simulink model "LPV_PitchControl_TwrFA_CP_Demonstrator_Integrator_TSR"  (R2018a)
settings: Solver=FixedStepAuto  StartTime=0.0  StopTime=TMax  FixedStep=Simulation.DT  RelTol=1e-3  EnableMultiTasking=on
undefined symbols (not defined in the file or in its folder): OutList, Parameters, rpm2radps, Simulation, strmatch
libraries: dspstat3 x4, simulink_extras x1
(part 1 of 2)
settings Model: ExtModeTrigMode=oneshot  ExtModeArmWhenConnect=off  Creator=Dana Martin  LastModifiedBy=dmartin
settings DataIOCC: SaveFormat=Array  SaveOutput=off  InspectSignalLogs=on  SignalLoggingName=sigsOut  OutputTimes=[0:500]/50
settings OptimizationCC: BooleanDataType=off  ExpressionDepthLimit=2147483647  InitFltsAndDblsToZero=on  LifeSpan=inf
settings DebuggingCC: SignalRangeChecking=warning  AlgebraicLoopMsg=error  SaveWithParameterizedLinksMsg=none  UnderspecifiedInitializationDetection=Classic  MergeDetectMultiDrivingBlocksExec=none  SignalResolutionControl=TryResolveAllWithWarning  TimeAdjustmentMsg=warning  MultiTaskDSMMsg=warning  MultiTaskCondExecSysMsg=warning  ParameterUnderflowMsg=warning  UnderSpecifiedDataTypeMsg=warning  UnnecessaryDatatypeConvMsg=warning  VectorMatrixConversionMsg=warning  FcnCallInpInsideContextMsg=warning  SignalLabelMismatchMsg=warning  SFcnCompatibilityMsg=warning  UniqueDataStoreMsg=warning  AllowSymbolicDim=off  ModelReferenceIOMsg=warning  ModelReferenceVersionMismatchMessage=warning  ModelReferenceIOMismatchMessage=warning  StateNameClashWarn=warning  StrictBusMsg=WarnOnBusTreatedAsVector  NonBusSignalsTreatedAsBus=warning  SFUnexpectedBacktrackingDiag=warning  SFNoUnconditionalDefaultTransitionDiag=warning  SFExecutionAtInitializationDiag=none
settings HardwareCC: ProdBitPerPointer=32  ProdBitPerSizeT=32  ProdBitPerPtrDiffT=32  ProdLargestAtomicFloat=None  ProdIntDivRoundTo=Undefined  ProdEndianess=Unspecified  ProdWordSize=32  ProdHWDeviceType=32-bit Generic  TargetBitPerPointer=64  TargetBitPerSizeT=64  TargetBitPerPtrDiffT=64  TargetLongLongMode=on  TargetIntDivRoundTo=Zero  TargetEndianess=LittleEndian  TargetWordSize=64  TargetHWDeviceType=MATLAB Host  ProdEqTarget=off
settings ModelReferenceCC: PropagateSignalLabelsOutOfModel=off
settings CodeAppCC: StateflowObjectComments=on
settings GRTTargetCC: TargetFcnLib=ansi_tfl_tmw.mat  TargetLangStandard=C89/C90 (ANSI)  ModelReferenceCompliant=off  GeneratePreprocessorConditionals=Disable all  CombineOutputUpdateFcns=off  GRTInterface=on
settings ConfigComp: CovMetricSettings=dw  CovHtmlReporting=on  CovSaveCumulativeToWorkspaceVar=on  CovSaveSingleToWorkspaceVar=on  CovExternalEMLEnable=off  CovSFcnEnable=off

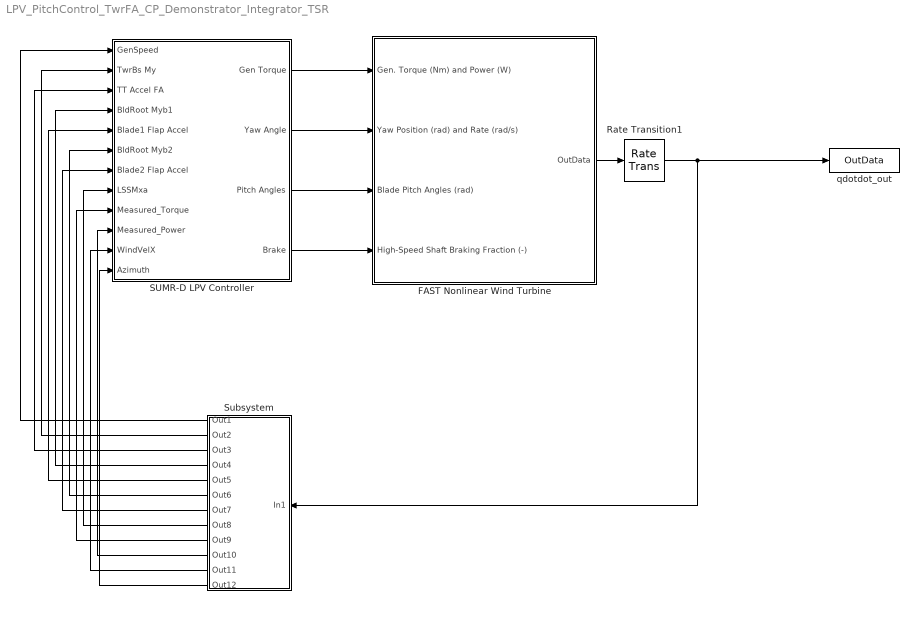
== system LPV_PitchControl_TwrFA_CP_Demonstrator_Integrator_TSR ==
  FAST Nonlinear Wind Turbine : Subsystem  mask(FAST Nonlinear Wind Turbine){}
      mask help: This block contains the FAST S-Function.
      mask init:
      | clear FAST_SFunc
  Rate Transition1 : RateTransition
  SUMR-D LPV Controller : Subsystem
  Subsystem : Subsystem
  qdotdot_out : ToWorkspace  VariableName=OutData  SaveFormat=Structure With Time  SampleTime=-1
  wires:
  SUMR-D LPV Controller/1(Gen Torque) -> FAST Nonlinear Wind Turbine/1(Gen. Torque (Nm) and Power (W))
  SUMR-D LPV Controller/3(Pitch Angles) -> FAST Nonlinear Wind Turbine/3(Blade Pitch Angles (rad))
  SUMR-D LPV Controller/2(Yaw Angle) -> FAST Nonlinear Wind Turbine/2(Yaw Position (rad) and Rate (rad/s))
  SUMR-D LPV Controller/4(Brake) -> FAST Nonlinear Wind Turbine/4(High-Speed Shaft Braking Fraction (-))
  Rate Transition1/1 -> Subsystem/1(In1), qdotdot_out/1
  FAST Nonlinear Wind Turbine/1(OutData) -> Rate Transition1/1
  Subsystem/1(Out1) -> SUMR-D LPV Controller/1(GenSpeed)
  Subsystem/2(Out2) -> SUMR-D LPV Controller/2(TwrBs My)
  Subsystem/3(Out3) -> SUMR-D LPV Controller/3(TT Accel FA)
  Subsystem/4(Out4) -> SUMR-D LPV Controller/4(BldRoot Myb1)
  Subsystem/5(Out5) -> SUMR-D LPV Controller/5(Blade1 Flap Accel)
  Subsystem/6(Out6) -> SUMR-D LPV Controller/6(BldRoot Myb2)
  Subsystem/7(Out7) -> SUMR-D LPV Controller/7(Blade2 Flap Accel)
  Subsystem/8(Out8) -> SUMR-D LPV Controller/8(LSSMxa)
  Subsystem/9(Out9) -> SUMR-D LPV Controller/9(Measured_Torque)
  Subsystem/10(Out10) -> SUMR-D LPV Controller/10(Measured_Power)
  Subsystem/11(Out11) -> SUMR-D LPV Controller/11(WindVelX)
  Subsystem/12(Out12) -> SUMR-D LPV Controller/12(Azimuth)

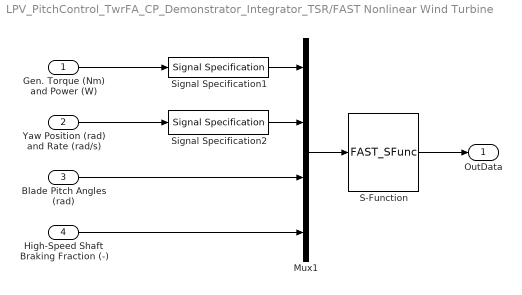
== system LPV_PitchControl_TwrFA_CP_Demonstrator_Integrator_TSR/FAST Nonlinear Wind Turbine ==
  Gen. Torque (Nm) and Power (W) : Inport
  Yaw Position (rad) and Rate (rad/s) : Inport  Port=2
  Blade Pitch Angles (rad) : Inport  Port=3
  High-Speed Shaft Braking Fraction (-) : Inport  Port=4
  Mux1 : Mux
  S-Function : S-Function  FunctionName=FAST_SFunc  Parameters=FAST_InputFileName, TMax, 0  SFunctionDeploymentMode=off  EnableBusSupport=off
  Signal Specification1 : SignalSpecification  OutDataTypeStr=double  Dimensions=2
  Signal Specification2 : SignalSpecification  OutDataTypeStr=double  Dimensions=2
  OutData : Outport
  wires:
  Gen. Torque (Nm) and Power (W)/1 -> Signal Specification1/1
  S-Function/1 -> OutData/1
  Mux1/1 -> S-Function/1
  Blade Pitch Angles (rad)/1 -> Mux1/3
  Yaw Position (rad) and Rate (rad/s)/1 -> Signal Specification2/1
  Signal Specification1/1 -> Mux1/1
  Signal Specification2/1 -> Mux1/2
  High-Speed Shaft Braking Fraction (-)/1 -> Mux1/4

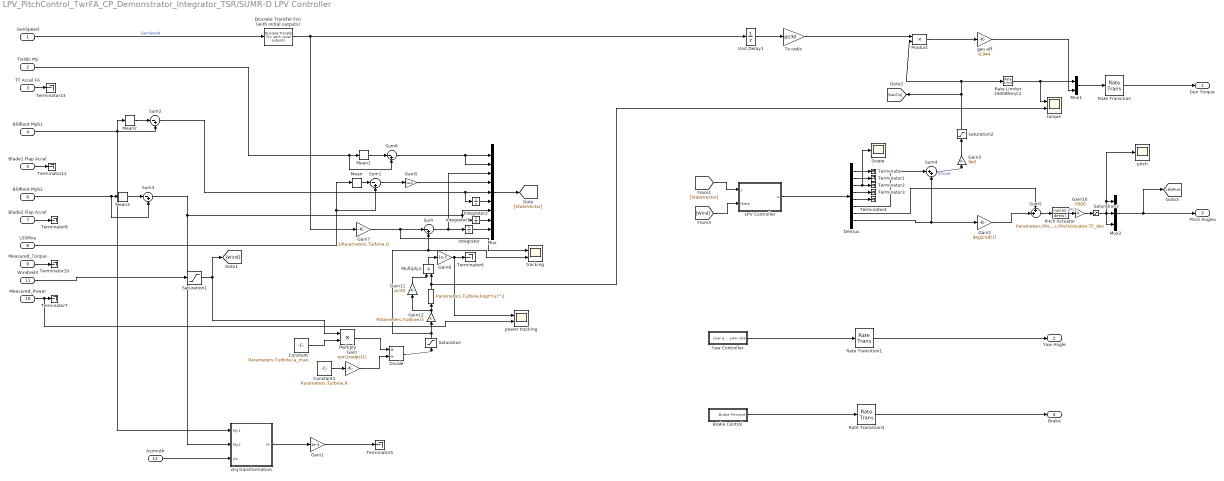
== system LPV_PitchControl_TwrFA_CP_Demonstrator_Integrator_TSR/SUMR-D LPV Controller ==
  GenSpeed : Inport
  TwrBs My : Inport  Port=2
  TT Accel FA : Inport  Port=3
  BldRoot Myb1 : Inport  Port=4
  Blade1 Flap Accel : Inport  Port=5
  BldRoot Myb2 : Inport  Port=6
  Blade2 Flap Accel : Inport  Port=7
  LSSMxa : Inport  Port=8
  Measured_Torque : Inport  Port=9
  Measured_Power : Inport  Port=10
  WindVelX : Inport  Port=11
  Azimuth : Inport  Port=12
  " " : Fcn  Expr=Parameters.Turbine.kopt*(u)^2
  Brake Control : Subsystem
  Constant : Constant  Value=Parameters.Turbine.la_max  SampleTime=Simulation.DT
  Constant1 : Constant  Value=Parameters.Turbine.R
  Demux : Demux  Outputs=8
  Discrete Transfer Fcn (with initial outputs) : simulink_extras/Additional Discrete/Discrete Transfer Fcn (with initial outputs)  N=Parameters.LPF.LPnum  D=Parameters.LPF.LPden  U0=Parameters.Turbine.IC.Wg  Y0=Parameters.Turbine.IC.Wg  TS=Simulation.DT
      settings: SourceProductName=Simulink  SourceProductBaseCode=SL
  Divide : Product  Inputs=*/
  Gain : Gain  Gain=rpm2radps(1)
  Gain1 : Gain  Gain=1e-3
  Gain10 : Gain  Gain=-5000
  Gain11 : Gain  Gain=pi/30
  Gain12 : Gain  Gain=Parameters.Turbine.G
  Gain2 : Gain  Gain=deg2rad(1)
  Gain3 : Gain  Gain=9e5
  Gain5 : Gain  Gain=1e-2
  Gain7 : Gain  Gain=1/Parameters.Turbine.G
  Gain8 : Gain  Gain=1e-3
  Integrator : Integrator
  Integrator1 : Integrator
  Integrator2 : Integrator
  LPV Controller : Subsystem  TreatAsAtomicUnit=on
      settings: MinAlgLoopOccurrences=on
  Mean{,1..3} (4 alike) : dspstat3/Mean  run=off  InputProcessing=Columns as channels (frame based)  reset_popup=None  directionMode=Each column  dimension=1  roiEnable=off  roiType=Rectangles  roiPortion=Entire ROI  roiOutput=Individual statistics for each ROI  roiFlag=off  roundingMode=Floor  overflowMode=off  outputDataTypeStr=Inherit: Same as accumulator  outputMin=[]  outputMax=[]  outputLastDataTypeStr=Inherit: Same as accumulator
  Multiply : Product
  Multiply1 : Product
  Mux : Mux  Inputs=9
  Mux1 : Mux  Inputs=2
  Mux2 : Mux  Inputs=3
  Pitch Actuator : TransferFcn  Numerator=Parameters.PitchActuator.TF_num  Denominator=Parameters.PitchActuator.TF_den
  Product : Product  RndMeth=Zero
  Rate Limiter 15000Nm/s1 : RateLimiter  RisingSlewLimit=15000  FallingSlewLimit=-15000  SampleTimeMode=inherited
  Rate Transition : RateTransition  InitialCondition=Parameters.Turbine.IC.Tg
  Rate Transition1 : RateTransition
  Rate Transition3 : RateTransition
  Saturation : Saturate  UpperLimit=Parameters.Turbine.wr_rated  LowerLimit=0
  Saturation1 : Saturate  UpperLimit=12  LowerLimit=0
  Saturation2 : Saturate  UpperLimit=Parameters.Turbine.T_rated  LowerLimit=-Parameters.Turbine.T_rated
  Saturation3 : Saturate  UpperLimit=deg2rad(90)  LowerLimit=deg2rad(Parameters.Turbine.fine_pitch)
  Scope : Scope
  Sum{,1..3,6} (5 alike) : Sum  Inputs=|-+
  Sum4 : Sum  Inputs=|++
  Sum5 : Sum  Inputs=++|
  Terminator{,1..8,10,12..13} (12 alike) : Terminator
  To rad/s : Gain  Gain=pi/30
  Unit Delay1 : UnitDelay  InitialCondition=Parameters.Turbine.IC.Wg  SampleTime=Simulation.DT
  Yaw Controller : Subsystem
  d-q transformation : MATLAB Function  TreatAsAtomicUnit=on
  gen eff : Gain  Gain=0.944
  pitch : Scope
  power tracking : Scope  NumInputPorts=2
  torque : Scope  NumInputPorts=2
  tracking : Scope  NumInputPorts=2
  Gen Torque : Outport
  Yaw Angle : Outport  Port=2
  Pitch Angles : Outport  Port=3
  Brake : Outport  Port=4
  wires:
  Mux1/1 -> Rate Transition/1
  Product/1 -> gen eff/1
  Unit Delay1/1 -> To rad/s/1
  To rad/s/1 -> Product/1
  gen eff/1 -> Mux1/2
  GenSpeed/1 -> Discrete Transfer Fcn (with initial outputs)/1  "GenSpeed"
  Yaw Controller/1(yaw and yaw rate) -> Rate Transition1/1
  Brake Control/1(Brake Percent) -> Rate Transition3/1
  Rate Transition3/1 -> Brake/1
  Rate Transition1/1 -> Yaw Angle/1
  Mux/1 -> [StateVector]
  [StateVector] -> LPV Controller/1(y)
  Demux/1 -> Terminator/1
  Demux/5 -> Terminator4/1
  LSSMxa/1 -> Sum1/2, Mean/1
  Mean/1 -> Sum1/1
  Constant/1 -> Multiply/2
  Multiply/1 -> Divide/1
  Constant1/1 -> Gain/1
  Gain/1 -> Divide/2
  Measured_Torque/1 -> Terminator10/1
  Azimuth/1 -> d-q transformation/3(Az)
  TT Accel FA/1 -> Terminator13/1
  LPV Controller/1(u) -> Demux/1
  Demux/2 -> Terminator1/1
  Demux/4 -> Terminator3/1
  Demux/3 -> Scope/1, Terminator2/1
  Mux2/1 -> [BldPitch], Pitch Angles/1
  Demux/7 -> Sum5/1
  Sum4/1 -> Gain3/1  "torque"
  Sum5/1 -> Pitch Actuator/1
  Integrator/1 -> Mux/9
  Gain2/1 -> Sum5/2
  Gain5/1 -> Mux/4
  Demux/8 -> Sum4/2, Gain2/1
  Rate Transition/1 -> Gen Torque/1
  Sum1/1 -> Gain5/1
  d-q transformation/1(M) -> Gain1/1
  Gain1/1 -> Terminator5/1
  [Wind] -> LPV Controller/2(theta)
  WindVelX/1 -> Saturation1/1
  Mean1/1 -> Sum6/1
  BldRoot Myb1/1 -> d-q transformation/1(My1), Mean2/1, Sum2/2
  Discrete Transfer Fcn (with initial outputs)/1 -> Gain7/1, Unit Delay1/1
  Demux/6 -> Sum4/1
  Mean2/1 -> Sum2/1
  Mean3/1 -> Sum3/1
  BldRoot Myb2/1 -> Sum3/2, Mean3/1
  TwrBs My/1 -> Sum6/2, Mean1/1
  Pitch Actuator/1 -> Gain10/1  "pitch"
  Saturation/1 -> Gain12/1, Sum/2, tracking/2
  Multiply1/1 -> Gain8/1
  Gain11/1 -> Multiply1/1
  " "/1 -> torque/2, Multiply1/2
  Divide/1 -> Saturation/1
  Gain12/1 -> Gain11/1, " "/1
  Gain8/1 -> power tracking/1, Terminator6/1
  Saturation1/1 -> [Wind], Multiply/1
  Measured_Power/1 -> power tracking/2, Terminator7/1
  Integrator2/1 -> Mux/6
  Integrator1/1 -> Mux/8
  Blade1 Flap Accel/1 -> Terminator12/1
  Blade2 Flap Accel/1 -> Terminator8/1
  Sum6/1 -> Mux/2, Mux/1
  Gain7/1 -> Sum/1, tracking/1
  Sum3/1 -> Mux/7, Integrator1/1, d-q transformation/2(My2)
  Sum2/1 -> Integrator2/1, Mux/5
  Gain10/1 -> Saturation3/1
  Saturation3/1 -> Mux2/3, Mux2/1, pitch/1, Mux2/2
  Sum/1 -> Mux/3, Integrator/1
  Rate Limiter 15000Nm/s1/1 -> Mux1/1, torque/1
  Saturation2/1 -> Product/2, Rate Limiter 15000Nm/s1/1, [GenTrq]
  Gain3/1 -> Saturation2/1

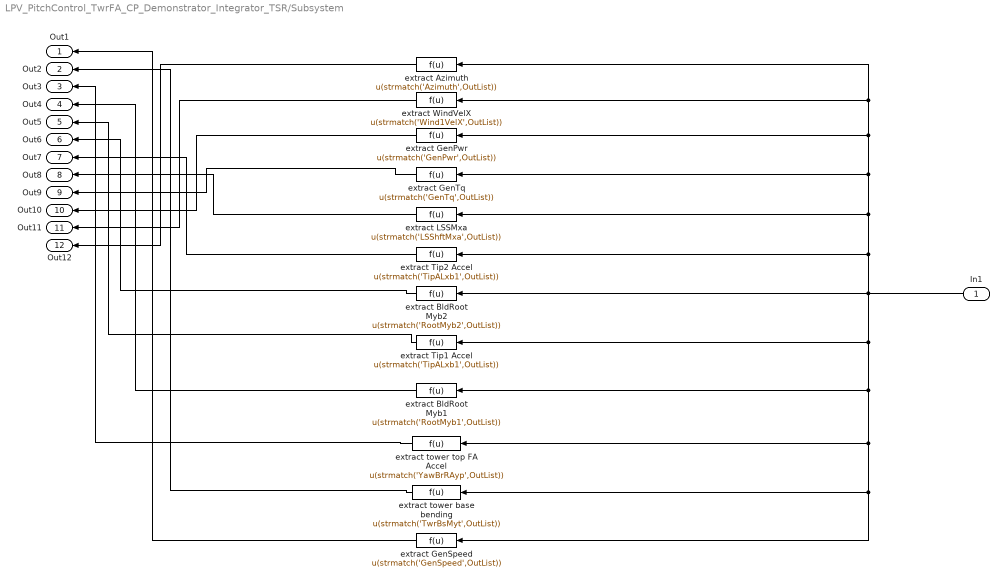
== system LPV_PitchControl_TwrFA_CP_Demonstrator_Integrator_TSR/Subsystem ==
  In1 : Inport
  extract Azimuth : Fcn  Expr=u(strmatch('Azimuth',OutList))
  extract BldRoot Myb1 : Fcn  Expr=u(strmatch('RootMyb1',OutList))
  extract BldRoot Myb2 : Fcn  Expr=u(strmatch('RootMyb2',OutList))
  extract GenPwr : Fcn  Expr=u(strmatch('GenPwr',OutList))
  extract GenSpeed : Fcn  Expr=u(strmatch('GenSpeed',OutList))
  extract GenTq : Fcn  Expr=u(strmatch('GenTq',OutList))
  extract LSSMxa : Fcn  Expr=u(strmatch('LSShftMxa',OutList))
  extract Tip1 Accel : Fcn  Expr=u(strmatch('TipALxb1',OutList))
  extract Tip2 Accel : Fcn  Expr=u(strmatch('TipALxb1',OutList))
  extract WindVelX : Fcn  Expr=u(strmatch('Wind1VelX',OutList))
  extract tower base bending : Fcn  Expr=u(strmatch('TwrBsMyt',OutList))
  extract tower top FA Accel : Fcn  Expr=u(strmatch('YawBrRAyp',OutList))
  Out1 : Outport
  Out2 : Outport  Port=2
  Out3 : Outport  Port=3
  Out4 : Outport  Port=4
  Out5 : Outport  Port=5
  Out6 : Outport  Port=6
  Out7 : Outport  Port=7
  Out8 : Outport  Port=8
  Out9 : Outport  Port=9
  Out10 : Outport  Port=10
  Out11 : Outport  Port=11
  Out12 : Outport  Port=12
  wires:
  extract WindVelX/1 -> Out11/1
  extract GenTq/1 -> Out9/1
  In1/1 -> extract Azimuth/1, extract WindVelX/1, extract GenPwr/1, extract GenTq/1, extract LSSMxa/1, extract Tip2 Accel/1, extract BldRoot Myb2/1, extract Tip1 Accel/1, extract BldRoot Myb1/1, extract tower base bending/1, extract GenSpeed/1, extract tower top FA Accel/1
  extract GenPwr/1 -> Out10/1
  extract Tip1 Accel/1 -> Out5/1
  extract LSSMxa/1 -> Out8/1
  extract tower base bending/1 -> Out2/1
  extract tower top FA Accel/1 -> Out3/1
  extract Tip2 Accel/1 -> Out7/1
  extract Azimuth/1 -> Out12/1
  extract BldRoot Myb2/1 -> Out6/1
  extract GenSpeed/1 -> Out1/1
  extract BldRoot Myb1/1 -> Out4/1

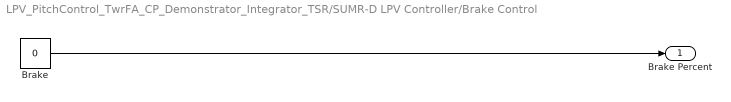
== system LPV_PitchControl_TwrFA_CP_Demonstrator_Integrator_TSR/SUMR-D LPV Controller/Brake Control ==
  Brake : Constant  Value=0  SampleTime=-1
  Brake Percent : Outport
  wires:
  Brake/1 -> Brake Percent/1

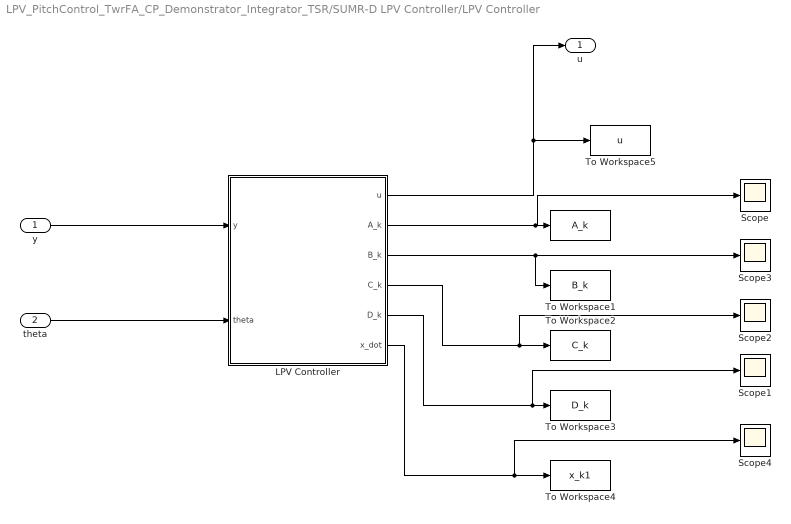
== system LPV_PitchControl_TwrFA_CP_Demonstrator_Integrator_TSR/SUMR-D LPV Controller/LPV Controller ==
  y : Inport
  theta : Inport  Port=2
  " " : ToWorkspace  VariableName=A_k  SaveFormat=Structure With Time  SampleTime=-1
      settings: Decimation=3
  LPV Controller : MATLAB Function  TreatAsAtomicUnit=on  SystemSampleTime=Simulation.DT
      settings: MinAlgLoopOccurrences=on
  Scope{,1..4} (5 alike) : Scope
  To Workspace1 : ToWorkspace  VariableName=B_k  SaveFormat=Structure With Time  SampleTime=-1
      settings: Decimation=3
  To Workspace2 : ToWorkspace  VariableName=C_k  SaveFormat=Structure With Time  SampleTime=-1
      settings: Decimation=3
  To Workspace3 : ToWorkspace  VariableName=D_k  SaveFormat=Structure With Time  SampleTime=-1
      settings: Decimation=3
  To Workspace4 : ToWorkspace  VariableName=x_k1  SaveFormat=Structure With Time  SampleTime=-1
      settings: Decimation=3
  To Workspace5 : ToWorkspace  VariableName=u  SaveFormat=Structure With Time  SampleTime=-1
      settings: Decimation=3
  u : Outport
  wires:
  theta/1 -> LPV Controller/2(theta)
  y/1 -> LPV Controller/1(y)
  LPV Controller/3(B_k) -> Scope3/1, To Workspace1/1
  LPV Controller/2(A_k) -> Scope/1, " "/1
  LPV Controller/5(D_k) -> Scope1/1, To Workspace3/1
  LPV Controller/1(u) -> To Workspace5/1, u/1
  LPV Controller/4(C_k) -> Scope2/1, To Workspace2/1
  LPV Controller/6(x_dot) -> Scope4/1, To Workspace4/1

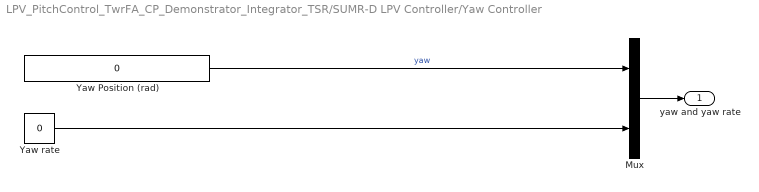
== system LPV_PitchControl_TwrFA_CP_Demonstrator_Integrator_TSR/SUMR-D LPV Controller/Yaw Controller ==
  Mux : Mux  Inputs=2
  Yaw Position (rad) : Constant  Value=0  SampleTime=-1
  Yaw rate : Constant  Value=0  SampleTime=-1
  yaw and yaw rate : Outport
  wires:
  Mux/1 -> yaw and yaw rate/1
  Yaw Position (rad)/1 -> Mux/1  "yaw"
  Yaw rate/1 -> Mux/2
